simulink model "Simple_Wiper_control_state"  (R2024a)
settings: Solver=VariableStepAuto  StartTime=0.0  StopTime=10.0  RelTol=1e-3
settings Model: Creator=DELL  LastModifiedBy=DELL

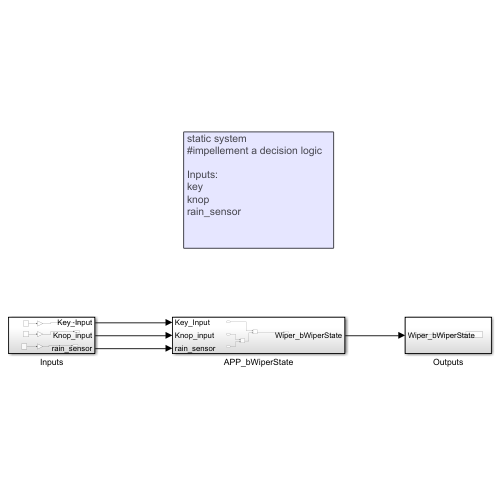
[thumbnail: Simulink's stored preview of the top-level diagram]
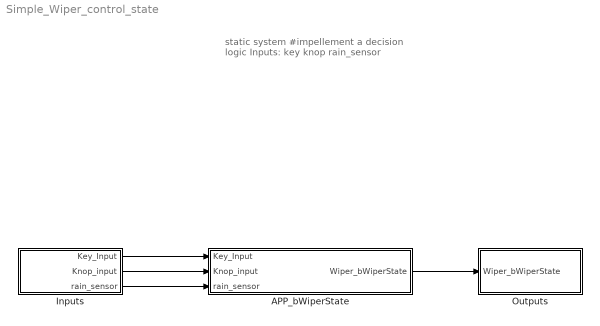
== system Simple_Wiper_control_state ==
  note: static system
      | #impellement a decision logic
      |
      | Inputs:
      | key
      | knop
      | rain_sensor
  APP_bWiperState : Subsystem
  Inputs : Subsystem
  Outputs : Subsystem
  wires:
  APP_bWiperState/1(Wiper_bWiperState) -> Outputs/1(Wiper_bWiperState)
  Inputs/1(Key_Input) -> APP_bWiperState/1(Key_Input)
  Inputs/2(Knop_input) -> APP_bWiperState/2(Knop_input)
  Inputs/3(rain_sensor) -> APP_bWiperState/3(rain_sensor)

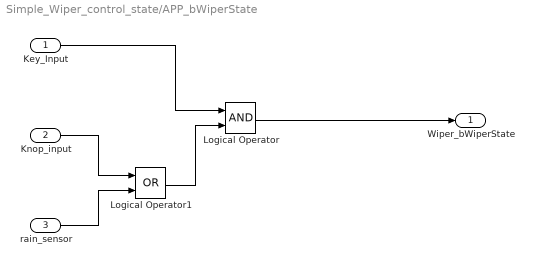
== system Simple_Wiper_control_state/APP_bWiperState ==
  Key_Input : Inport
  Knop_input : Inport  Port=2
  rain_sensor : Inport  Port=3
  Logical Operator : Logic  AllPortsSameDT=off  OutDataTypeStr=boolean
  Logical Operator1 : Logic  Operator=OR  AllPortsSameDT=off  OutDataTypeStr=boolean
  Wiper_bWiperState : Outport
  wires:
  Knop_input/1 -> Logical Operator1/1
  rain_sensor/1 -> Logical Operator1/2
  Logical Operator1/1 -> Logical Operator/2
  Key_Input/1 -> Logical Operator/1
  Logical Operator/1 -> Wiper_bWiperState/1

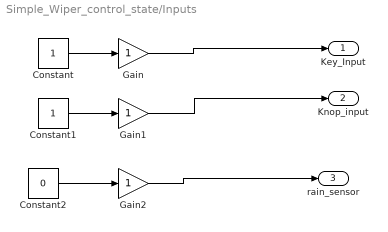
== system Simple_Wiper_control_state/Inputs ==
  Constant : Constant
  Constant1 : Constant
  Constant2 : Constant  Value=0
  Gain : Gain
  Gain1 : Gain
  Gain2 : Gain
  Key_Input : Outport
  Knop_input : Outport  Port=2
  rain_sensor : Outport  Port=3
  wires:
  Constant/1 -> Gain/1
  Constant1/1 -> Gain1/1
  Constant2/1 -> Gain2/1
  Gain/1 -> Key_Input/1
  Gain1/1 -> Knop_input/1
  Gain2/1 -> rain_sensor/1

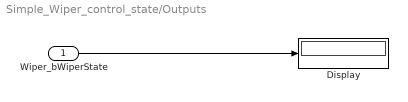
== system Simple_Wiper_control_state/Outputs ==
  Wiper_bWiperState : Inport
  Display : Display
  wires:
  Wiper_bWiperState/1 -> Display/1
